simulink model "Test"  (R2018b)
settings: Solver=VariableStepAuto  StartTime=0.0  StopTime=10.0  MaxStep=0.001  MinStep=0.0001  RelTol=1e-3
model workspace (MAT data in the model file):
  Ball.radius = 0.03
  Ball.density = 1000
  Plane.length = 1
  Plane.width = 1
  Plane.depth = 0.1
  SCARA_Robot = robotics.RigidBodyTree
  SCARA_Robot.TreeInternal = robotics.manip.internal.RigidBodyTree
  SCARA_Robot.TreeInternal.NumBodies = 7
  SCARA_Robot.TreeInternal.Base = robotics.manip.internal.RigidBody
  SCARA_Robot.TreeInternal.Base.Index = 0
  SCARA_Robot.TreeInternal.Base.NameInternal = 'Base'
  SCARA_Robot.TreeInternal.Base.JointInternal = robotics.Joint
  SCARA_Robot.TreeInternal.Base.JointInternal.Type = 'fixed'
  SCARA_Robot.TreeInternal.Base.JointInternal.VelocityNumber = 0
  SCARA_Robot.TreeInternal.Base.JointInternal.PositionNumber = 0
  SCARA_Robot.TreeInternal.Base.JointInternal.MotionSubspace = [0; 0; 0; 0; 0; 0]
  SCARA_Robot.TreeInternal.Base.JointInternal.NameInternal = 'base_jnt'
  SCARA_Robot.TreeInternal.Base.ParentIndex = -1
  SCARA_Robot.TreeInternal.Base.ChildrenIndices = [1 0 0 0 0 0 1]
  SCARA_Robot.TreeInternal.Base.MassInternal = 1
  SCARA_Robot.TreeInternal.Base.CenterOfMassInternal = [0 0 0]
  SCARA_Robot.TreeInternal.Base.InertiaInternal = [1  0  0; 0  1  0; 0  0  1]
  SCARA_Robot.TreeInternal.Base.SpatialInertia = [1  0  0  0  0  0; 0  1  0  0  0  0; 0  0  1  0  0  0; 0  0  0  1  0  0; 0  0  0  0  1  0; 0  0  0  0  0  1]
  SCARA_Robot.TreeInternal.Gravity = [0 0 -9.80665]
  SCARA_Robot.TreeInternal.Bodies{1} = robotics.manip.internal.RigidBody
  SCARA_Robot.TreeInternal.Bodies{1}.Index = 1
  SCARA_Robot.TreeInternal.Bodies{1}.NameInternal = 'Body1'
  SCARA_Robot.TreeInternal.Bodies{1}.JointInternal = robotics.Joint
  SCARA_Robot.TreeInternal.Bodies{1}.JointInternal.Type = 'revolute'
  SCARA_Robot.TreeInternal.Bodies{1}.JointInternal.VelocityNumber = 1
  SCARA_Robot.TreeInternal.Bodies{1}.JointInternal.PositionNumber = 1
  SCARA_Robot.TreeInternal.Bodies{1}.JointInternal.MotionSubspace = [0; 0; 1; 0; 0; 0]
  SCARA_Robot.TreeInternal.Bodies{1}.JointInternal.InTree = 1
  SCARA_Robot.TreeInternal.Bodies{1}.JointInternal.JointToParentTransform = [1  0  0  0; 0  1  0  0; 0  0  1  0.2335; 0  0  0  1]
  SCARA_Robot.TreeInternal.Bodies{1}.JointInternal.NameInternal = 'Joint1'
  SCARA_Robot.TreeInternal.Bodies{1}.JointInternal.PositionLimitsInternal = [-3.14159265359 3.14159265359]
  SCARA_Robot.TreeInternal.Bodies{1}.JointInternal.JointAxisInternal = [0 0 1]
  SCARA_Robot.TreeInternal.Bodies{1}.ParentIndex = 0
  SCARA_Robot.TreeInternal.Bodies{1}.ChildrenIndices = [0 1]
  SCARA_Robot.TreeInternal.Bodies{1}.MassInternal = 3.12934702863
  SCARA_Robot.TreeInternal.Bodies{1}.CenterOfMassInternal = [0.108937389495 0 0.0763962080079]
  SCARA_Robot.TreeInternal.Bodies{1}.InertiaInternal = [0.0248122549552  -1.93363586828e-20  -0.0276846659585; -1.93363586828e-20  0.092692509819  4.00877355014e-19; -0.0276846659585  4.00877355014e-19  0.0776265146367]
  SCARA_Robot.TreeInternal.Bodies{1}.SpatialInertia = [0.0248122549552  -1.93363586828e-20  -0.0276846659585  0  -0.239070246528  0; -1.93363586828e-20  0.092692509819  4.00877355014e-19  0.239070246528  0  -0.340902896122; -0.0276846659585  4.00877355014e-19  0.0776265146367  0  0.340902896122  0; 0  0.239070246528  0  3.12934702863  0  0; -0.239070246528  0  0.340902896122  0  3.12934702863  0; 0  -0.340902896122  0  0  0  3.12934702863]
  SCARA_Robot.TreeInternal.Bodies{2} = robotics.manip.internal.RigidBody
  SCARA_Robot.TreeInternal.Bodies{2}.Index = 2
  SCARA_Robot.TreeInternal.Bodies{2}.NameInternal = 'Body2'
  SCARA_Robot.TreeInternal.Bodies{2}.JointInternal = robotics.Joint
  SCARA_Robot.TreeInternal.Bodies{2}.JointInternal.Type = 'revolute'
  SCARA_Robot.TreeInternal.Bodies{2}.JointInternal.VelocityNumber = 1
  SCARA_Robot.TreeInternal.Bodies{2}.JointInternal.PositionNumber = 1
  SCARA_Robot.TreeInternal.Bodies{2}.JointInternal.MotionSubspace = [0; 0; 1; 0; 0; 0]
  SCARA_Robot.TreeInternal.Bodies{2}.JointInternal.InTree = 1
  SCARA_Robot.TreeInternal.Bodies{2}.JointInternal.JointToParentTransform = [1  0  0  0.25; 0  1  0  0; 0  0  1  0.09; 0  0  0  1]
  SCARA_Robot.TreeInternal.Bodies{2}.JointInternal.NameInternal = 'Joint2'
  SCARA_Robot.TreeInternal.Bodies{2}.JointInternal.PositionLimitsInternal = [-3.14159265359 3.14159265359]
  SCARA_Robot.TreeInternal.Bodies{2}.JointInternal.JointAxisInternal = [0 0 1]
  SCARA_Robot.TreeInternal.Bodies{2}.ParentIndex = 1
  SCARA_Robot.TreeInternal.Bodies{2}.ChildrenIndices = [0 0 1]
  SCARA_Robot.TreeInternal.Bodies{2}.MassInternal = 2.8
  SCARA_Robot.TreeInternal.Bodies{2}.CenterOfMassInternal = [0.0730251626831 0 0.08]
  SCARA_Robot.TreeInternal.Bodies{2}.InertiaInternal = [0.0343024465413  9.77217250727e-20  -0.016902140627; 9.77217250727e-20  0.0618863054598  -9.17919345749e-19; -0.016902140627  -9.17919345749e-19  0.0363706015866]
  SCARA_Robot.TreeInternal.Bodies{2}.SpatialInertia = [0.0343024465413  9.77217250727e-20  -0.016902140627  0  -0.224  0; 9.77217250727e-20  0.0618863054598  -9.17919345749e-19  0.224  0  -0.204470455513; -0.016902140627  -9.17919345749e-19  0.0363706015866  0  0.204470455513  0; 0  0.224  0  2.8  0  0; -0.224  0  0.204470455513  0  2.8  0; 0  -0.204470455513  0  0  0  2.8]
  SCARA_Robot.TreeInternal.Bodies{3} = robotics.manip.internal.RigidBody
  SCARA_Robot.TreeInternal.Bodies{3}.Index = 3
  SCARA_Robot.TreeInternal.Bodies{3}.NameInternal = 'Body3'
  SCARA_Robot.TreeInternal.Bodies{3}.JointInternal = robotics.Joint
  SCARA_Robot.TreeInternal.Bodies{3}.JointInternal.Type = 'prismatic'
  SCARA_Robot.TreeInternal.Bodies{3}.JointInternal.VelocityNumber = 1
  SCARA_Robot.TreeInternal.Bodies{3}.JointInternal.PositionNumber = 1
  SCARA_Robot.TreeInternal.Bodies{3}.JointInternal.MotionSubspace = [0; 0; 0; 0; 0; 1]
  SCARA_Robot.TreeInternal.Bodies{3}.JointInternal.InTree = 1
  SCARA_Robot.TreeInternal.Bodies{3}.JointInternal.JointToParentTransform = [1  0  0  0.142; 0  1  0  -0.008; 0  0  1  0.25; 0  0  0  1]
  SCARA_Robot.TreeInternal.Bodies{3}.JointInternal.NameInternal = 'Joint3'
  SCARA_Robot.TreeInternal.Bodies{3}.JointInternal.PositionLimitsInternal = [-0.5 0.5]
  SCARA_Robot.TreeInternal.Bodies{3}.JointInternal.JointAxisInternal = [0 0 1]
  SCARA_Robot.TreeInternal.Bodies{3}.ParentIndex = 2
  SCARA_Robot.TreeInternal.Bodies{3}.ChildrenIndices = [0 0 0 1]
  SCARA_Robot.TreeInternal.Bodies{3}.MassInternal = 0.0658123859659
  SCARA_Robot.TreeInternal.Bodies{3}.CenterOfMassInternal = [0.008 0.008 -0.161652320553]
  SCARA_Robot.TreeInternal.Bodies{3}.InertiaInternal = [0.00223249562485  -4.21199270182e-06  8.51097993001e-05; -4.21199270182e-06  0.00223249562485  8.51097993001e-05; 8.51097993001e-05  8.51097993001e-05  1.08030484212e-05]
  SCARA_Robot.TreeInternal.Bodies{3}.SpatialInertia = [0.00223249562485  -4.21199270182e-06  8.51097993001e-05  0  0.0106387249125  0.000526499087728; -4.21199270182e-06  0.00223249562485  8.51097993001e-05  -0.0106387249125  0  -0.000526499087728; 8.51097993001e-05  8.51097993001e-05  1.08030484212e-05  -0.000526499087728  0.000526499087728  0; 0  -0.0106387249125  -0.000526499087728  0.0658123859659  0  0; 0.0106387249125  0  0.000526499087728  0  0.0658123859659  0; 0.000526499087728  -0.000526499087728  0  0  0  0.0658123859659]
  SCARA_Robot.TreeInternal.Bodies{4} = robotics.manip.internal.RigidBody
  SCARA_Robot.TreeInternal.Bodies{4}.Index = 4
  SCARA_Robot.TreeInternal.Bodies{4}.NameInternal = 'Body4'
  SCARA_Robot.TreeInternal.Bodies{4}.JointInternal = robotics.Joint
  SCARA_Robot.TreeInternal.Bodies{4}.JointInternal.Type = 'revolute'
  SCARA_Robot.TreeInternal.Bodies{4}.JointInternal.VelocityNumber = 1
  SCARA_Robot.TreeInternal.Bodies{4}.JointInternal.PositionNumber = 1
  SCARA_Robot.TreeInternal.Bodies{4}.JointInternal.MotionSubspace = [0; 0; 1; 0; 0; 0]
  SCARA_Robot.TreeInternal.Bodies{4}.JointInternal.InTree = 1
  SCARA_Robot.TreeInternal.Bodies{4}.JointInternal.JointToParentTransform = [1  0  0  0.008; 0  1  0  0.008; 0  0  1  -0.02; 0  0  0  1]
  SCARA_Robot.TreeInternal.Bodies{4}.JointInternal.NameInternal = 'Joint4'
  SCARA_Robot.TreeInternal.Bodies{4}.JointInternal.PositionLimitsInternal = [-3.14159265359 3.14159265359]
  SCARA_Robot.TreeInternal.Bodies{4}.JointInternal.JointAxisInternal = [0 0 1]
  SCARA_Robot.TreeInternal.Bodies{4}.ParentIndex = 3
  SCARA_Robot.TreeInternal.Bodies{4}.ChildrenIndices = [0 0 0 0 1]
  SCARA_Robot.TreeInternal.Bodies{4}.MassInternal = 0.0638828919245
  SCARA_Robot.TreeInternal.Bodies{4}.CenterOfMassInternal = [-0.000115977158264 0 -0.314685264828]
  SCARA_Robot.TreeInternal.Bodies{4}.InertiaInternal = [0.00634242429346  0  -2.33382122413e-06; 0  0.0063422366579  0; -2.33382122413e-06  0  2.29864595889e-05]
  SCARA_Robot.TreeInternal.Bodies{4}.SpatialInertia = [0.00634242429346  0  -2.33382122413e-06  0  0.0201030047632  0; 0  0.0063422366579  0  -0.0201030047632  0  7.40895626708e-06; -2.33382122413e-06  0  2.29864595889e-05  0  -7.40895626708e-06  0; 0  -0.0201030047632  0  0.0638828919245  0  0; 0.0201030047632  0  -7.40895626708e-06  0  0.0638828919245  0; 0  7.40895626708e-06  0  0  0  0.0638828919245]
  SCARA_Robot.TreeInternal.Bodies{5} = robotics.manip.internal.RigidBody
  SCARA_Robot.TreeInternal.Bodies{5}.Index = 5
  SCARA_Robot.TreeInternal.Bodies{5}.NameInternal = 'Body5'
  SCARA_Robot.TreeInternal.Bodies{5}.JointInternal = robotics.Joint
  SCARA_Robot.TreeInternal.Bodies{5}.JointInternal.Type = 'fixed'
  SCARA_Robot.TreeInternal.Bodies{5}.JointInternal.VelocityNumber = 0
  SCARA_Robot.TreeInternal.Bodies{5}.JointInternal.PositionNumber = 0
  SCARA_Robot.TreeInternal.Bodies{5}.JointInternal.MotionSubspace = [0; 0; 0; 0; 0; 0]
  SCARA_Robot.TreeInternal.Bodies{5}.JointInternal.InTree = 1
  SCARA_Robot.TreeInternal.Bodies{5}.JointInternal.JointToParentTransform = [1  0  0  -2.71050543121e-20; 0  1  0  0; 0  0  1  -0.33; 0  0  0  1]
  SCARA_Robot.TreeInternal.Bodies{5}.JointInternal.NameInternal = 'Joint5'
  SCARA_Robot.TreeInternal.Bodies{5}.ParentIndex = 4
  SCARA_Robot.TreeInternal.Bodies{5}.ChildrenIndices = [0 0 0 0 0 1]
  SCARA_Robot.TreeInternal.Bodies{5}.MassInternal = 0
  SCARA_Robot.TreeInternal.Bodies{5}.CenterOfMassInternal = [0 0 0]
  SCARA_Robot.TreeInternal.Bodies{5}.InertiaInternal = [0  0  0; 0  0  0; 0  0  0]
  SCARA_Robot.TreeInternal.Bodies{5}.SpatialInertia = [0  0  0  0  0  0; 0  0  0  0  0  0; 0  0  0  0  0  0; 0  0  0  0  0  0; 0  0  0  0  0  0; 0  0  0  0  0  0]
  SCARA_Robot.TreeInternal.Bodies{6} = robotics.manip.internal.RigidBody
  SCARA_Robot.TreeInternal.Bodies{6}.Index = 6
  SCARA_Robot.TreeInternal.Bodies{6}.NameInternal = 'Body6'
  SCARA_Robot.TreeInternal.Bodies{6}.JointInternal = robotics.Joint
  SCARA_Robot.TreeInternal.Bodies{6}.JointInternal.Type = 'fixed'
  SCARA_Robot.TreeInternal.Bodies{6}.JointInternal.VelocityNumber = 0
  SCARA_Robot.TreeInternal.Bodies{6}.JointInternal.PositionNumber = 0
  SCARA_Robot.TreeInternal.Bodies{6}.JointInternal.MotionSubspace = [0; 0; 0; 0; 0; 0]
  SCARA_Robot.TreeInternal.Bodies{6}.JointInternal.InTree = 1
  SCARA_Robot.TreeInternal.Bodies{6}.JointInternal.JointToParentTransform = [1  0  0  0; 0  1  0  0; 0  0  1  0; 0  0  0  1]
  SCARA_Robot.TreeInternal.Bodies{6}.JointInternal.NameInternal = 'Joint6'
  SCARA_Robot.TreeInternal.Bodies{6}.ParentIndex = 5
  SCARA_Robot.TreeInternal.Bodies{6}.ChildrenIndices = [0 0 0 0 0]
  SCARA_Robot.TreeInternal.Bodies{6}.MassInternal = 0.113097335529
  SCARA_Robot.TreeInternal.Bodies{6}.CenterOfMassInternal = [0 0 0]
  SCARA_Robot.TreeInternal.Bodies{6}.InertiaInternal = [4.07150407905e-05  0  0; 0  4.07150407905e-05  0; 0  0  4.07150407905e-05]
  SCARA_Robot.TreeInternal.Bodies{6}.SpatialInertia = [4.07150407905e-05  0  0  0  0  0; 0  4.07150407905e-05  0  0  0  0; 0  0  4.07150407905e-05  0  0  0; 0  0  0  0.113097335529  0  0; 0  0  0  0  0.113097335529  0; 0  0  0  0  0  0.113097335529]
  SCARA_Robot.TreeInternal.Bodies{7} = robotics.manip.internal.RigidBody
  SCARA_Robot.TreeInternal.Bodies{7}.Index = 7
  SCARA_Robot.TreeInternal.Bodies{7}.NameInternal = 'Body7'
  SCARA_Robot.TreeInternal.Bodies{7}.JointInternal = robotics.Joint
  SCARA_Robot.TreeInternal.Bodies{7}.JointInternal.Type = 'fixed'
  SCARA_Robot.TreeInternal.Bodies{7}.JointInternal.VelocityNumber = 0
  SCARA_Robot.TreeInternal.Bodies{7}.JointInternal.PositionNumber = 0
  SCARA_Robot.TreeInternal.Bodies{7}.JointInternal.MotionSubspace = [0; 0; 0; 0; 0; 0]
  SCARA_Robot.TreeInternal.Bodies{7}.JointInternal.InTree = 1
  SCARA_Robot.TreeInternal.Bodies{7}.JointInternal.JointToParentTransform = [1  0  0  0; 0  1  0  0; 0  0  1  0; 0  0  0  1]
  SCARA_Robot.TreeInternal.Bodies{7}.JointInternal.NameInternal = 'Joint7'
  SCARA_Robot.TreeInternal.Bodies{7}.ParentIndex = 0
  SCARA_Robot.TreeInternal.Bodies{7}.ChildrenIndices = [0 0 0 0 0 0]
  SCARA_Robot.TreeInternal.Bodies{7}.MassInternal = 0
  SCARA_Robot.TreeInternal.Bodies{7}.CenterOfMassInternal = [0 0 0]
  SCARA_Robot.TreeInternal.Bodies{7}.InertiaInternal = [0  0  0; 0  0  0; 0  0  0]
  SCARA_Robot.TreeInternal.Bodies{7}.SpatialInertia = [0  0  0  0  0  0; 0  0  0  0  0  0; 0  0  0  0  0  0; 0  0  0  0  0  0; 0  0  0  0  0  0; 0  0  0  0  0  0]
  SCARA_Robot.TreeInternal.NumNonFixedBodies = 4
  SCARA_Robot.TreeInternal.PositionNumber = 4
  SCARA_Robot.TreeInternal.VelocityNumber = 4
  SCARA_Robot.TreeInternal.PositionDoFMap = [1  1; 2  2; 3  3; 4  4; 0  -1; 0  -1; 0  -1]
  SCARA_Robot.TreeInternal.VelocityDoFMap = [1  1; 2  2; 3  3; 4  4; 0  -1; 0  -1; 0  -1]
  SCARA_Robot.TreeInternal.MaxNumBodies = 7
  SCARA_Robot.TreeInternal.MaxNameLength = 200
  SCARA_Robot.TreeInternal.MaxJointPositionNumber = 7
  SCARA_Robot.TreeInternal.VisualizationInfo = robotics.manip.internal.VisualizationInfo
  SCARA_Robot.TreeInternal.VisualizationInfo.ShowTag = 'DO_NOT_EDIT_DRLYM'
  SCARA_Robot.TreeInternal.DataFormatInternal = 'struct'
  Sig = Simulink.Signal
  Sig.DataType = 'auto'
  Sig.Dimensions = -1
  Sig.DimensionsMode = 'auto'
  Sig.Complexity = 'auto'
  Sig.SampleTime = -1
  Sig.SamplingMode = 'auto'
  smiData.RigidTransform(1).translation = [250 0 20]
  smiData.RigidTransform(1).angle = 3.14159265359
  smiData.RigidTransform(1).axis = [1 0 0]
  smiData.RigidTransform(1).ID = 'B[Link1-1:-:Link2-1]'
  smiData.RigidTransform(2).translation = [0 0 270]
  smiData.RigidTransform(2).angle = 3.14159265359
  smiData.RigidTransform(2).axis = [1 0 0]
  smiData.RigidTransform(2).ID = 'F[Link1-1:-:Link2-1]'
  smiData.RigidTransform(3).translation = [0 0 110]
  smiData.RigidTransform(3).angle = 0
  smiData.RigidTransform(3).axis = [0 0 0]
  smiData.RigidTransform(3).ID = 'B[Base-1:-:Link1-1]'
  smiData.RigidTransform(4).translation = [0 0 110]
  smiData.RigidTransform(4).angle = 3.14159265359
  smiData.RigidTransform(4).axis = [1 0 0]
  smiData.RigidTransform(4).ID = 'F[Base-1:-:Link1-1]'
  smiData.RigidTransform(5).translation = [142 8 20]
  smiData.RigidTransform(5).angle = 3.14159265359
  smiData.RigidTransform(5).axis = [1 0 0]
  smiData.RigidTransform(5).ID = 'B[Link2-1:-:Move-1]'
  smiData.RigidTransform(6).translation = [-8 -8 320]
  smiData.RigidTransform(6).angle = 0
  smiData.RigidTransform(6).axis = [0 0 1]
  smiData.RigidTransform(6).ID = 'F[Link2-1:-:Move-1]'
  smiData.RigidTransform(7).translation = [0 0 300]
  smiData.RigidTransform(7).angle = 3.14159265359
  smiData.RigidTransform(7).axis = [1 0 0]
  smiData.RigidTransform(7).ID = 'B[Move-1:-:Rot-1]'
  smiData.RigidTransform(8).translation = [0 0 -300]
  smiData.RigidTransform(8).angle = 0
  smiData.RigidTransform(8).axis = [0 0 0]
  smiData.RigidTransform(8).ID = 'F[Move-1:-:Rot-1]'
  smiData.RigidTransform(9).translation = [0 0 123.5]
  smiData.RigidTransform(9).angle = 0
  smiData.RigidTransform(9).axis = [0 0 0]
  smiData.RigidTransform(9).ID = 'RootGround[Base-1]'
  smiData.Solid(1).mass = 2.8
  smiData.Solid(1).CoM = [73.0251626831 0 190]
  smiData.Solid(1).MoI = [16382.4465413 29034.8171821 21439.1133089]
  smiData.Solid(1).PoI = [0 544.504186027 0]
  smiData.Solid(1).color = [0.8 0.3 0.3]
  smiData.Solid(1).opacity = 1
  smiData.Solid(1).ID = 'Link2*:*榛樿'
  smiData.Solid(2).mass = 0.0638828919245
  smiData.Solid(2).CoM = [-0.115977158264 0 15.3147351721]
  smiData.Solid(2).MoI = [16.3049156988 16.1164208702 22.9856003192]
  smiData.Solid(2).PoI = [0 -0.00233185912567 0]
  smiData.Solid(2).color = [0.3 0.8 0.3]
  smiData.Solid(2).opacity = 1
  smiData.Solid(2).ID = 'Rot*:*榛樿'
  smiData.Solid(3).mass = 7.54037730286
  smiData.Solid(3).CoM = [0 -12.2090965753 111.939248054]
  smiData.Solid(3).MoI = [67953.4260367 46975.8188154 47346.1777637]
  smiData.Solid(3).PoI = [2150.03105694 0 0]
  smiData.Solid(3).color = [1 0.5 0.8]
  smiData.Solid(3).opacity = 1
  smiData.Solid(3).ID = 'Base*:*榛樿'
  smiData.Solid(4).mass = 3.12934702863
  smiData.Solid(4).CoM = [108.937389495 0 33.6037919921]
  smiData.Solid(4).MoI = [6548.19467291 37291.3779621 40489.4430621]
  smiData.Solid(4).PoI = [0 1640.97739592 0]
  smiData.Solid(4).color = [0.3 0.3 0.5]
  smiData.Solid(4).opacity = 1
  smiData.Solid(4).ID = 'Link1*:*榛樿'
  smiData.Solid(5).mass = 0.0658123859659
  smiData.Solid(5).CoM = [0 0 158.347679447]
  smiData.Solid(5).MoI = [508.509062318 508.509062318 2.37906301758]
  smiData.Solid(5).PoI = [0 0 0]
  smiData.Solid(5).color = [1 0.3 0.3]
  smiData.Solid(5).opacity = 1
  smiData.Solid(5).ID = 'Move*:*榛樿'
  smiData.PrismaticJoint.Pz.Pos = 0
  smiData.PrismaticJoint.ID = '[Link2-1:-:Move-1]'
  smiData.RevoluteJoint(1).Rz.Pos = 0
  smiData.RevoluteJoint(1).ID = '[Link1-1:-:Link2-1]'
  smiData.RevoluteJoint(2).Rz.Pos = 0
  smiData.RevoluteJoint(2).ID = '[Base-1:-:Link1-1]'
  smiData.RevoluteJoint(3).Rz.Pos = 0
  smiData.RevoluteJoint(3).ID = '[Move-1:-:Rot-1]'
values from neighbouring files (symbols this model uses):
  smiData = struct    [SCARA_Robot_DataFile.m]
undefined symbols (not defined in the file or in its folder): X, Y, Z
libraries: sm_lib x35, nesl_utility x17, robotmaniplib x6
settings Model: Creator=wqq  LastModifiedBy=wqq

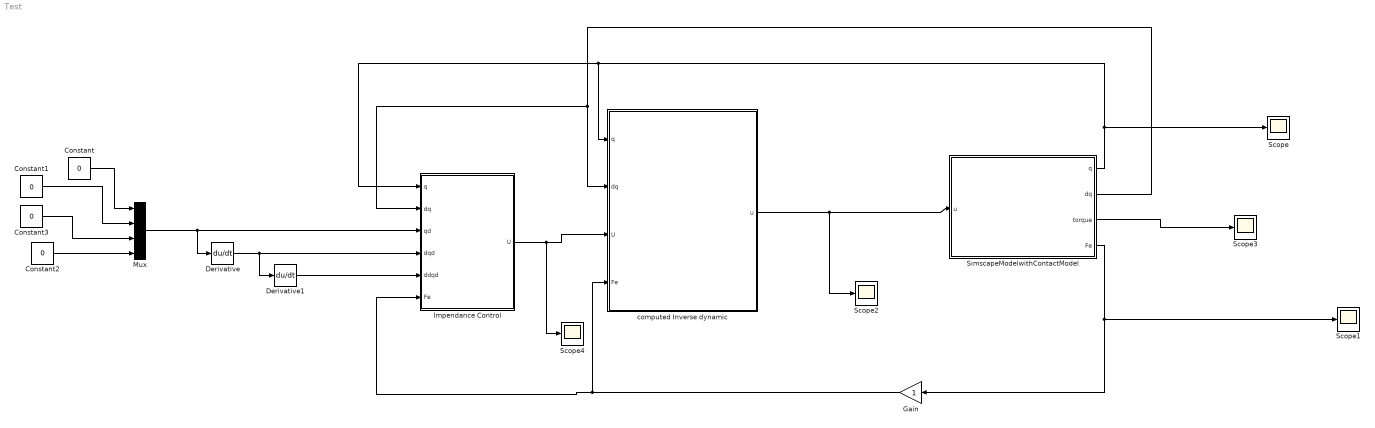
== system Test ==
  Constant{,1..3} (4 alike) : Constant  Value=0
  Derivative : Derivative
  Derivative1 : Derivative
  Gain : Gain
  Impendance Control : Subsystem
  Mux : Mux
  Scope{,1..4} (5 alike) : Scope
  SimscapeModelwithContactModel : Subsystem
  computed Inverse dynamic : Subsystem
  wires:
  SimscapeModelwithContactModel/2(dq) -> computed Inverse dynamic/2(dq), Impendance Control/2(dq)
  SimscapeModelwithContactModel/1(q) -> Scope/1, computed Inverse dynamic/1(q), Impendance Control/1(q)
  Mux/1 -> Derivative/1, Impendance Control/3(qd)
  Constant1/1 -> Mux/2
  Constant/1 -> Mux/1
  SimscapeModelwithContactModel/3(torque) -> Scope3/1
  Derivative1/1 -> Impendance Control/5(ddqd)
  SimscapeModelwithContactModel/4(Fe) -> Scope1/1, Gain/1
  Gain/1 -> computed Inverse dynamic/4(Fe), Impendance Control/6(Fe)
  Constant3/1 -> Mux/3
  computed Inverse dynamic/1(u) -> Scope2/1, SimscapeModelwithContactModel/1(u)
  Derivative/1 -> Derivative1/1, Impendance Control/4(dqd)
  Impendance Control/1(U) -> Scope4/1, computed Inverse dynamic/3(U)
  Constant2/1 -> Mux/4

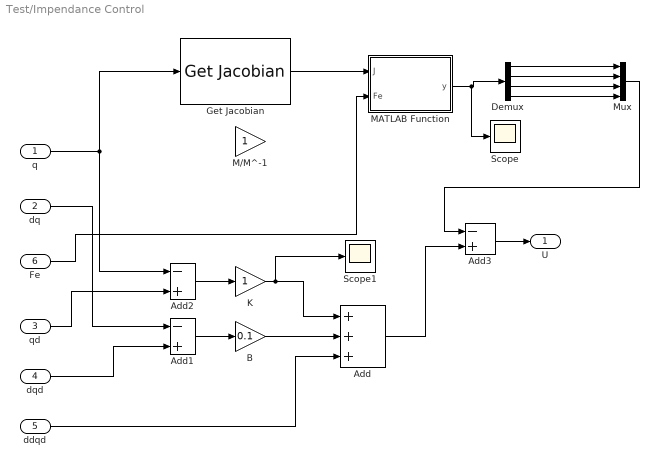
== system Test/Impendance Control ==
  q : Inport
  dq : Inport  Port=2
  qd : Inport  Port=3
  dqd : Inport  Port=4
  ddqd : Inport  Port=5
  Fe : Inport  Port=6
  Add : Sum  Inputs=+++
  Add1 : Sum  Inputs=-+
  Add2 : Sum  Inputs=-+
  Add3 : Sum  Inputs=-+
  B : Gain  Gain=0.1
  Demux : Demux
  Get Jacobian : robotmaniplib/Get Jacobian  RigidBodyTree=SCARA_Robot  EndEffector=Body7
      settings: SourceProductName=Robotics System Toolbox
  K : Gain
  M/M^-1 : Gain
  MATLAB Function : MATLAB Function  TreatAsAtomicUnit=on
  Mux : Mux
  Scope : Scope
  Scope1 : Scope
  U : Outport
  wires:
  ddqd/1 -> Add/3
  dqd/1 -> Add1/2
  dq/1 -> Add1/1
  Add1/1 -> B/1
  B/1 -> Add/2
  qd/1 -> Add2/2
  Add2/1 -> K/1
  K/1 -> Scope1/1, Add/1
  Add/1 -> Add3/2
  Add3/1 -> U/1
  q/1 -> Add2/1, Get Jacobian/1
  Get Jacobian/1 -> MATLAB Function/1(J)
  Fe/1 -> MATLAB Function/2(Fe)
  MATLAB Function/1(y) -> Scope/1, Demux/1
  Demux/1 -> Mux/1
  Demux/2 -> Mux/2
  Demux/3 -> Mux/3
  Demux/4 -> Mux/4
  Mux/1 -> Add3/1

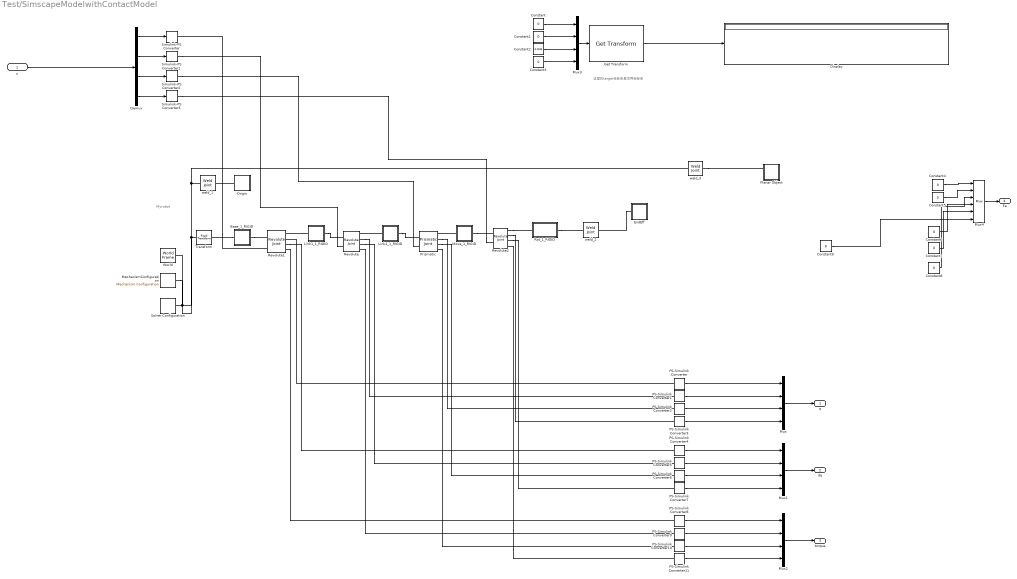
== system Test/SimscapeModelwithContactModel ==
  note: 这里的target坐标系是世界坐标系
  note: Myrobot
  u : Inport
  Base_1_RIGID : Subsystem
  Constant{,1,3..9} (9 alike) : Constant  Value=0
  Constant2 : Constant  Value=-0.2235
  Demux : Demux
  Display : Display
  EndEff : Subsystem
  Get Transform : robotmaniplib/Get Transform  RigidBodyTree=SCARA_Robot  SourceBody=Body5  TargetBody=Body7
      settings: SourceProductName=Robotics System Toolbox
  Link1_1_RIGID : Subsystem
  Link2_1_RIGID : Subsystem
  MechanismConfiguration : sm_lib/Utilities/Mechanism Configuration  UniformGravity=Constant  GravityVector=[0 0 -9.80665]  GravityUnits=m/s^2  LinearizationDelta=0.001
  Move_1_RIGID : Subsystem
  Mux{,1..3} (4 alike) : Mux
  Mux4 : Mux  Inputs=6
  Origin : Subsystem
  PS-Simulink Converter{,1..11} (12 alike) : nesl_utility/PS-Simulink Converter  PhysicalDomain=network_engine_domain  SubClassName=ps_output  LeftPortType=input  RightPortType=output  PseudoPeriodic=off  Frequencies=[]  Unit=1  AffineConversion=off
  Planar Object : Subsystem
  Prismatic : sm_lib/Joints/Prismatic Joint  SenseConstraintForce=off  SenseConstraintForceX=off  SenseConstraintForceY=off  SenseConstraintForceZ=off  SenseConstraintTorque=off  SenseConstraintTorqueX=off  SenseConstraintTorqueY=off  SenseConstraintTorqueZ=off  SenseTotalForce=off  SenseTotalForceX=off  SenseTotalForceY=off  SenseTotalForceZ=off  SenseTotalTorque=off  SenseTotalTorqueX=off  SenseTotalTorqueY=off  SenseTotalTorqueZ=off  CompositeWrenchDir=FollowerOnBase  CompositeWrenchFrame=BaseFrame  EquilibriumPosition=0  EquilibriumPositionUnits=m  SpringStiffness=0  SpringStiffnessUnits=N/m  DampingCoefficient=0  DampingCoefficientUnits=N/(m/s)  TorqueActuationMode=InputTorque  MotionActuationMode=ComputedMotion  SensePosition=on  SenseVelocity=on  SenseAcceleration=off  SenseTorqueForce=on  PositionTargetSpecify=on  PositionTargetPriority=High  PositionTargetValue=smiData.PrismaticJoint(1).Pz.Pos  PositionTargetValueUnits=m  VelocityTargetSpecify=off  VelocityTargetPriority=High  VelocityTargetValue=0  VelocityTargetValueUnits=m/s
  Revolute : sm_lib/Joints/Revolute Joint  SenseConstraintForce=off  SenseConstraintForceX=off  SenseConstraintForceY=off  SenseConstraintForceZ=off  SenseConstraintTorque=off  SenseConstraintTorqueX=off  SenseConstraintTorqueY=off  SenseConstraintTorqueZ=off  SenseTotalForce=off  SenseTotalForceX=off  SenseTotalForceY=off  SenseTotalForceZ=off  SenseTotalTorque=off  SenseTotalTorqueX=off  SenseTotalTorqueY=off  SenseTotalTorqueZ=off  CompositeWrenchDir=FollowerOnBase  CompositeWrenchFrame=BaseFrame  EquilibriumPosition=0  EquilibriumPositionUnits=rad  SpringStiffness=0  SpringStiffnessUnits=N*m/rad  DampingCoefficient=0  DampingCoefficientUnits=N*m/(rad/s)  TorqueActuationMode=InputTorque  MotionActuationMode=ComputedMotion  SensePosition=on  SenseVelocity=on  SenseAcceleration=off  SenseTorqueForce=on  PositionTargetSpecify=on  PositionTargetPriority=High  PositionTargetValue=smiData.RevoluteJoint(1).Rz.Pos  PositionTargetValueUnits=deg  VelocityTargetSpecify=off  VelocityTargetPriority=High  VelocityTargetValue=0  VelocityTargetValueUnits=deg/s
  Revolute1 : sm_lib/Joints/Revolute Joint  SenseConstraintForce=off  SenseConstraintForceX=off  SenseConstraintForceY=off  SenseConstraintForceZ=off  SenseConstraintTorque=off  SenseConstraintTorqueX=off  SenseConstraintTorqueY=off  SenseConstraintTorqueZ=off  SenseTotalForce=off  SenseTotalForceX=off  SenseTotalForceY=off  SenseTotalForceZ=off  SenseTotalTorque=off  SenseTotalTorqueX=off  SenseTotalTorqueY=off  SenseTotalTorqueZ=off  CompositeWrenchDir=FollowerOnBase  CompositeWrenchFrame=BaseFrame  EquilibriumPosition=0  EquilibriumPositionUnits=rad  SpringStiffness=0  SpringStiffnessUnits=N*m/rad  DampingCoefficient=0  DampingCoefficientUnits=N*m/(rad/s)  TorqueActuationMode=InputTorque  MotionActuationMode=ComputedMotion  SensePosition=on  SenseVelocity=on  SenseAcceleration=off  SenseTorqueForce=on  PositionTargetSpecify=on  PositionTargetPriority=High  PositionTargetValue=smiData.RevoluteJoint(2).Rz.Pos  PositionTargetValueUnits=deg  VelocityTargetSpecify=off  VelocityTargetPriority=High  VelocityTargetValue=0  VelocityTargetValueUnits=deg/s
  Revolute2 : sm_lib/Joints/Revolute Joint  SenseConstraintForce=off  SenseConstraintForceX=off  SenseConstraintForceY=off  SenseConstraintForceZ=off  SenseConstraintTorque=off  SenseConstraintTorqueX=off  SenseConstraintTorqueY=off  SenseConstraintTorqueZ=off  SenseTotalForce=off  SenseTotalForceX=off  SenseTotalForceY=off  SenseTotalForceZ=off  SenseTotalTorque=off  SenseTotalTorqueX=off  SenseTotalTorqueY=off  SenseTotalTorqueZ=off  CompositeWrenchDir=FollowerOnBase  CompositeWrenchFrame=BaseFrame  EquilibriumPosition=0  EquilibriumPositionUnits=rad  SpringStiffness=0  SpringStiffnessUnits=N*m/rad  DampingCoefficient=0  DampingCoefficientUnits=N*m/(rad/s)  TorqueActuationMode=InputTorque  MotionActuationMode=ComputedMotion  SensePosition=on  SenseVelocity=on  SenseAcceleration=off  SenseTorqueForce=on  PositionTargetSpecify=on  PositionTargetPriority=High  PositionTargetValue=smiData.RevoluteJoint(3).Rz.Pos  PositionTargetValueUnits=deg  VelocityTargetSpecify=off  VelocityTargetPriority=High  VelocityTargetValue=0  VelocityTargetValueUnits=deg/s
  Rot_1_RIGID : Subsystem
  Simulink-PS Converter{,1..3} (4 alike) : nesl_utility/Simulink-PS Converter  PhysicalDomain=network_engine_domain  SubClassName=ps_input  LeftPortType=input  RightPortType=output  PseudoPeriodic=off  Frequencies=[]  NoiseDistribution=none  NoiseParameters=[]  Unit=1  AffineConversion=off  FilteringAndDerivatives=provide  SimscapeFilterOrder=1  InputFilterTimeConstant=0.001  UdotUserProvided=0
  Solver Configuration : nesl_utility/Solver Configuration  PhysicalDomain=network_engine_domain  SubClassName=solver  LeftPortType=input  RightPortType=generic  Tones=[]  Harmonics=[]  SimulateNoise=off  Profile=off  UseLocalSampling=off  EnableSwitchedLinearOptims=on  FrequencyDomain=off  UseCCode=off  RelTol=0.001  AbsTol=1e-06  MinStep=1e-09  ToWorkspace=off  RevertToSquareIcSolve=off  NumHomotopyIterations=100  PhasorMode=off  PhasorModeNumHarmonics=1  DoDC=off  ResidualTolerance=1e-09  UseLocalSolver=off  LocalSolverChoice=NE_BACKWARD_EULER_ADVANCER  LocalSolverSampleTime=0.001  DoFixedCost=off  MaxNonlinIter=3  MaxModeIter=2  LinearAlgebra=auto  EquationFormulation=NE_TIME_EF  DelaysMemoryBudget=1024  AutomaticFiltering=on  FilteringTimeConstant=0.001  PartitionStorageMethod=AS_NEEDED  PartitionMemoryBudget=1024
  Transform : sm_lib/Frames and Transforms/Rigid Transform  TranslationMethod=Cartesian  TranslationStandardOffset=0  TranslationLengthUnit=mm  TranslationStandardAxis=+Z  TranslationCartesianOffset=smiData.RigidTransform(9).translation  TranslationROffset=0  TranslationROffsetUnits=m  TranslationZOffset=0  TranslationZOffsetUnits=m  TranslationThetaOffset=0  TranslationThetaOffsetUnits=deg  RotationMethod=ArbitraryAxis  RotationAngleUnits=rad  RotationStandardAxis=+Z  RotationAngle=smiData.RigidTransform(9).angle  RotationArbitraryAxis=smiData.RigidTransform(9).axis  FollAlignAxisA=+X  BaseAlignAxisA=+Y  FollAlignAxisB=+Y  BaseAlignAxisB=+Z  RotationSequenceAxes=FollowerAxes  RotationSequence=XYX  RotationSequenceAngles=[0 0 0]  RotationSequenceAnglesUnits=deg  RotationMatrix=[1 0 0; 0 1 0; 0 0 1]
  World : sm_lib/Frames and Transforms/World Frame
  weld_1 : sm_lib/Joints/Weld Joint  SenseConstraintForce=off  SenseConstraintForceX=off  SenseConstraintForceY=off  SenseConstraintForceZ=off  SenseConstraintTorque=off  SenseConstraintTorqueX=off  SenseConstraintTorqueY=off  SenseConstraintTorqueZ=off  SenseTotalForce=off  SenseTotalForceX=off  SenseTotalForceY=off  SenseTotalForceZ=off  SenseTotalTorque=off  SenseTotalTorqueX=off  SenseTotalTorqueY=off  SenseTotalTorqueZ=off  CompositeWrenchDir=FollowerOnBase  CompositeWrenchFrame=BaseFrame
  weld_2 : sm_lib/Joints/Weld Joint  SenseConstraintForce=off  SenseConstraintForceX=off  SenseConstraintForceY=off  SenseConstraintForceZ=off  SenseConstraintTorque=off  SenseConstraintTorqueX=off  SenseConstraintTorqueY=off  SenseConstraintTorqueZ=off  SenseTotalForce=off  SenseTotalForceX=off  SenseTotalForceY=off  SenseTotalForceZ=off  SenseTotalTorque=off  SenseTotalTorqueX=off  SenseTotalTorqueY=off  SenseTotalTorqueZ=off  CompositeWrenchDir=FollowerOnBase  CompositeWrenchFrame=BaseFrame
  weld_3 : sm_lib/Joints/Weld Joint  SenseConstraintForce=off  SenseConstraintForceX=off  SenseConstraintForceY=off  SenseConstraintForceZ=off  SenseConstraintTorque=off  SenseConstraintTorqueX=off  SenseConstraintTorqueY=off  SenseConstraintTorqueZ=off  SenseTotalForce=off  SenseTotalForceX=off  SenseTotalForceY=off  SenseTotalForceZ=off  SenseTotalTorque=off  SenseTotalTorqueX=off  SenseTotalTorqueY=off  SenseTotalTorqueZ=off  CompositeWrenchDir=FollowerOnBase  CompositeWrenchFrame=BaseFrame
  q : Outport
  dq : Outport  Port=2
  torque : Outport  Port=3
  Fe : Outport  Port=4
  wires:
  Demux/4 -> Simulink-PS Converter3/1
  Mux1/1 -> dq/1
  PS-Simulink Converter10/1 -> Mux2/3
  PS-Simulink Converter8/1 -> Mux2/1
  Demux/3 -> Simulink-PS Converter2/1
  Demux/1 -> Simulink-PS Converter/1
  PS-Simulink Converter11/1 -> Mux2/4
  PS-Simulink Converter5/1 -> Mux1/2
  PS-Simulink Converter/1 -> Mux/1
  Mux2/1 -> torque/1
  PS-Simulink Converter1/1 -> Mux/2
  Demux/2 -> Simulink-PS Converter1/1
  PS-Simulink Converter9/1 -> Mux2/2
  PS-Simulink Converter6/1 -> Mux1/3
  PS-Simulink Converter7/1 -> Mux1/4
  PS-Simulink Converter4/1 -> Mux1/1
  Mux/1 -> q/1
  PS-Simulink Converter2/1 -> Mux/3
  PS-Simulink Converter3/1 -> Mux/4
  Mux3/1 -> Get Transform/1
  Constant/1 -> Mux3/1
  Constant1/1 -> Mux3/2
  Constant2/1 -> Mux3/3
  Constant3/1 -> Mux3/4
  u/1 -> Demux/1
  Get Transform/1 -> Display/1
  Constant4/1 -> Mux4/1
  Constant5/1 -> Mux4/2
  Mux4/1 -> Fe/1
  Constant6/1 -> Mux4/4
  Constant7/1 -> Mux4/5
  Constant8/1 -> Mux4/3
  Constant9/1 -> Mux4/6
  connections:
  Revolute2/RConn3 -- PS-Simulink Converter7/LConn1
  Revolute/RConn2 -- PS-Simulink Converter1/LConn1
  Link2_1_RIGID/LConn1 -- Revolute/RConn1
  Move_1_RIGID/LConn1 -- Prismatic/RConn1
  Link1_1_RIGID/LConn1 -- Revolute1/RConn1
  Base_1_RIGID/LConn1 -- Transform/RConn1
  Revolute2/RConn2 -- PS-Simulink Converter3/LConn1
  Revolute1/LConn2 -- Simulink-PS Converter/RConn1
  Revolute1/RConn3 -- PS-Simulink Converter4/LConn1
  Simulink-PS Converter3/RConn1 -- Revolute2/LConn2
  Revolute1/RConn4 -- PS-Simulink Converter8/LConn1
  Move_1_RIGID/RConn1 -- Revolute2/LConn1
  PS-Simulink Converter/LConn1 -- Revolute1/RConn2
  Revolute/RConn4 -- PS-Simulink Converter9/LConn1
  Link2_1_RIGID/RConn1 -- Prismatic/LConn1
  Base_1_RIGID/RConn1 -- Revolute1/LConn1
  Link1_1_RIGID/RConn1 -- Revolute/LConn1
  Revolute2/RConn1 -- Rot_1_RIGID/LConn1
  Prismatic/RConn2 -- PS-Simulink Converter2/LConn1
  Revolute2/RConn4 -- PS-Simulink Converter11/LConn1
  Simulink-PS Converter2/RConn1 -- Prismatic/LConn2
  Simulink-PS Converter1/RConn1 -- Revolute/LConn2
  Revolute/RConn3 -- PS-Simulink Converter5/LConn1
  Prismatic/RConn3 -- PS-Simulink Converter6/LConn1
  Prismatic/RConn4 -- PS-Simulink Converter10/LConn1
  Rot_1_RIGID/RConn1 -- weld_2/LConn1
  EndEff/LConn1 -- weld_2/RConn1
  Origin/LConn1 -- weld_1/RConn1
  weld_1/LConn1 -- World/RConn1 -- MechanismConfiguration/RConn1 -- Solver Configuration/RConn1 -- Transform/LConn1 -- weld_3/LConn1
  weld_3/RConn1 -- Planar Object/LConn1

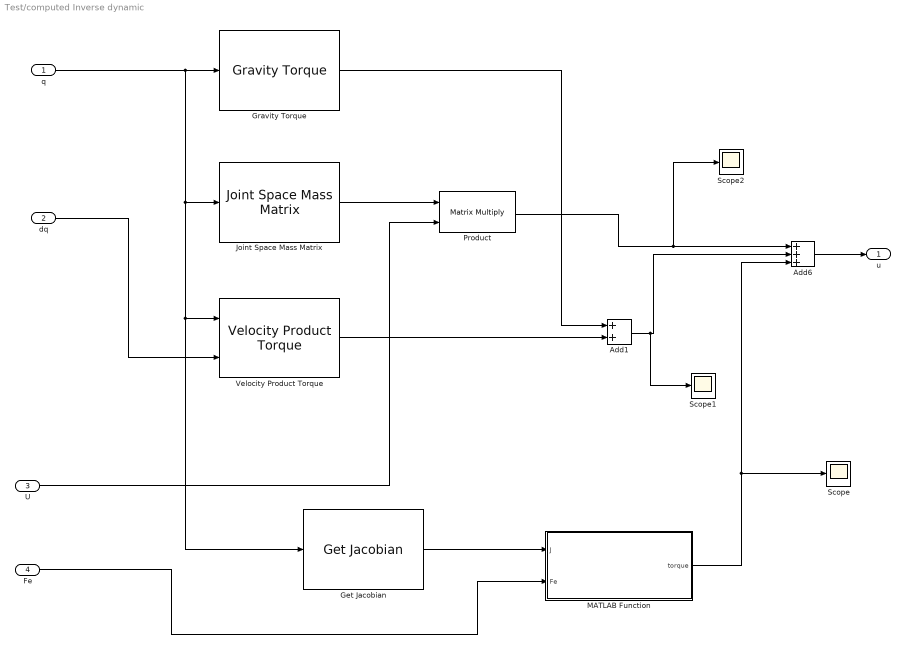
== system Test/computed Inverse dynamic ==
  q : Inport
  dq : Inport  Port=2
  U : Inport  Port=3
  Fe : Inport  Port=4
  Add1 : Sum
  Add6 : Sum  Inputs=+++
  Get Jacobian : robotmaniplib/Get Jacobian  RigidBodyTree=SCARA_Robot  EndEffector=Body7
      settings: SourceProductName=Robotics System Toolbox
  Gravity Torque : robotmaniplib/Gravity Torque  RigidBodyTree=SCARA_Robot
      settings: SourceProductName=Robotics System Toolbox
  Joint Space Mass Matrix : robotmaniplib/Joint Space Mass Matrix  RigidBodyTree=SCARA_Robot
      settings: SourceProductName=Robotics System Toolbox
  MATLAB Function : MATLAB Function  TreatAsAtomicUnit=on
  Product : Product  Multiplication=Matrix(*)
  Scope : Scope
  Scope1 : Scope
  Scope2 : Scope
  Velocity Product Torque : robotmaniplib/Velocity Product Torque  RigidBodyTree=SCARA_Robot
      settings: SourceProductName=Robotics System Toolbox
  u : Outport
  wires:
  q/1 -> Get Jacobian/1, Velocity Product Torque/1, Joint Space Mass Matrix/1, Gravity Torque/1
  dq/1 -> Velocity Product Torque/2
  Gravity Torque/1 -> Add1/1
  Joint Space Mass Matrix/1 -> Product/1
  Velocity Product Torque/1 -> Add1/2
  Add1/1 -> Scope1/1, Add6/2
  Product/1 -> Scope2/1, Add6/1
  Add6/1 -> u/1
  U/1 -> Product/2
  Get Jacobian/1 -> MATLAB Function/1(J)
  Fe/1 -> MATLAB Function/2(Fe)
  MATLAB Function/1(torque) -> Scope/1, Add6/3

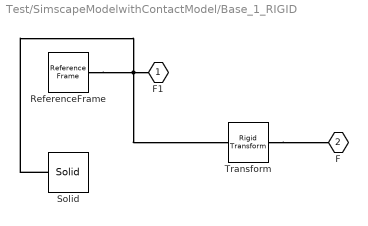
== system Test/SimscapeModelwithContactModel/Base_1_RIGID ==
  ReferenceFrame : sm_lib/Frames and Transforms/Reference Frame
  Solid : sm_lib/Body Elements/Solid  InertiaType=Custom  Mass=smiData.Solid(3).mass  MassUnits=kg  CenterOfMass=smiData.Solid(3).CoM  CenterOfMassUnits=mm  MomentsOfInertia=smiData.Solid(3).MoI  MomentsOfInertiaUnits=kg*mm^2  ProductsOfInertia=smiData.Solid(3).PoI  ProductsOfInertiaUnits=kg*mm^2  BasedOnType=Density  Density=1000  DensityUnits=kg/m^3  DoExposeReferenceFrame=off  SerializedFrames=<Frames><Frame><Id>Frame1</Id><Value><Name>F2</Name><Origin><Source>GeometricFeature</Source><FeatureName>cylindrical surface 2</FeatureName></Origin><PrimaryAxis><DefinedDirection>+Z</DefinedDirection><Source>ReferenceFrame</Source><SourceDirection>+Z</SourceDirection><FeatureName></FeatureName></PrimaryAxis><SecondaryAxis><DefinedDirection>+X</DefinedDirection><Source>ReferenceFrame</Source><SourceDirection>+X</SourceDirection><FeatureName></FeatureName></SecondaryAxis></Value></Frame></Frames>  GraphicType=FromGeometry  MarkerShape=Sphere  MarkerSize=10  GraphicVisPropType=SimpleVisualProperties  GraphicDiffuseColor=smiData.Solid(3).color  GraphicSpecularColor=[0.5 0.5 0.5 1.0]  GraphicAmbientColor=[0.15 0.15 0.15 1.0]  GraphicEmissiveColor=[0.0 0.0 0.0 1.0]  GraphicShininess=75  GraphicOpacity=smiData.Solid(3).opacity  GeometryShape=FromFile  RectangleSize=[1 1]  RectangleSizeUnits=m  BrickDimensions=[1 1 1]  BrickDimensionUnits=m  CylinderRadius=1  CylinderRadiusUnits=m  CylinderLength=1  CylinderLengthUnits=m  SphereRadius=1  SphereRadiusUnits=m  EllipsoidRadii=[1 1 1]  EllipsoidRadiiUnits=m  ExtrusionCrossSection=[1 1; -1 1; -1 -1; 1 -1]  ExtrusionCrossSectionUnits=m  ExtrusionLength=1  ExtrusionLengthUnits=m  PolygonNumSides=3  PolygonOuterRadius=1  PolygonOuterRadiusUnits=m  ExtGeomFileType=STEP  ExtGeomFileName=Base_默认_sldprt.STEP  ExtGeomFileUnits=m  RevolutionCrossSection=[1 1; 1 -1; 2 -1; 2 1]  RevolutionCrossSectionUnits=m  RevolutionExtent=Full  RevolutionAngle=180  RevolutionAngleUnits=deg
  Transform : sm_lib/Frames and Transforms/Rigid Transform  TranslationMethod=Cartesian  TranslationStandardOffset=0  TranslationLengthUnit=mm  TranslationStandardAxis=+Z  TranslationCartesianOffset=smiData.RigidTransform(3).translation  TranslationROffset=0  TranslationROffsetUnits=m  TranslationZOffset=0  TranslationZOffsetUnits=m  TranslationThetaOffset=0  TranslationThetaOffsetUnits=deg  RotationMethod=ArbitraryAxis  RotationAngleUnits=rad  RotationStandardAxis=+Z  RotationAngle=smiData.RigidTransform(3).angle  RotationArbitraryAxis=smiData.RigidTransform(3).axis  FollAlignAxisA=+X  BaseAlignAxisA=+Y  FollAlignAxisB=+Y  BaseAlignAxisB=+Z  RotationSequenceAxes=FollowerAxes  RotationSequence=XYX  RotationSequenceAngles=[0 0 0]  RotationSequenceAnglesUnits=deg  RotationMatrix=[1 0 0; 0 1 0; 0 0 1]
  F1 : PMIOPort  Side=Left
  F : PMIOPort  Port=2  Side=Right
  connections:
  ReferenceFrame/RConn1 -- Solid/LConn1 -- Transform/LConn1 -- F1/RConn1
  Transform/RConn1 -- F/RConn1

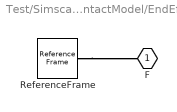
== system Test/SimscapeModelwithContactModel/EndEff ==
  ReferenceFrame : sm_lib/Frames and Transforms/Reference Frame
  F : PMIOPort  Side=Left
  connections:
  ReferenceFrame/RConn1 -- F/RConn1

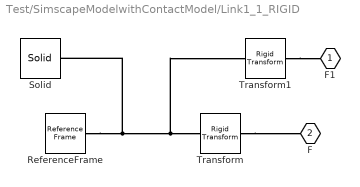
== system Test/SimscapeModelwithContactModel/Link1_1_RIGID ==
  ReferenceFrame : sm_lib/Frames and Transforms/Reference Frame
  Solid : sm_lib/Body Elements/Solid  InertiaType=Custom  Mass=smiData.Solid(4).mass  MassUnits=kg  CenterOfMass=smiData.Solid(4).CoM  CenterOfMassUnits=mm  MomentsOfInertia=smiData.Solid(4).MoI  MomentsOfInertiaUnits=kg*mm^2  ProductsOfInertia=smiData.Solid(4).PoI  ProductsOfInertiaUnits=kg*mm^2  BasedOnType=Density  Density=1000  DensityUnits=kg/m^3  DoExposeReferenceFrame=on  SerializedFrames=<Frames/>  GraphicType=FromGeometry  MarkerShape=Sphere  MarkerSize=10  GraphicVisPropType=SimpleVisualProperties  GraphicDiffuseColor=smiData.Solid(4).color  GraphicSpecularColor=[0.5 0.5 0.5 1.0]  GraphicAmbientColor=[0.15 0.15 0.15 1.0]  GraphicEmissiveColor=[0.0 0.0 0.0 1.0]  GraphicShininess=75  GraphicOpacity=smiData.Solid(4).opacity  GeometryShape=FromFile  RectangleSize=[1 1]  RectangleSizeUnits=m  BrickDimensions=[1 1 1]  BrickDimensionUnits=m  CylinderRadius=1  CylinderRadiusUnits=m  CylinderLength=1  CylinderLengthUnits=m  SphereRadius=1  SphereRadiusUnits=m  EllipsoidRadii=[1 1 1]  EllipsoidRadiiUnits=m  ExtrusionCrossSection=[1 1; -1 1; -1 -1; 1 -1]  ExtrusionCrossSectionUnits=m  ExtrusionLength=1  ExtrusionLengthUnits=m  PolygonNumSides=3  PolygonOuterRadius=1  PolygonOuterRadiusUnits=m  ExtGeomFileType=STEP  ExtGeomFileName=Link1_默认_sldprt.STEP  ExtGeomFileUnits=m  RevolutionCrossSection=[1 1; 1 -1; 2 -1; 2 1]  RevolutionCrossSectionUnits=m  RevolutionExtent=Full  RevolutionAngle=180  RevolutionAngleUnits=deg
  Transform : sm_lib/Frames and Transforms/Rigid Transform  TranslationMethod=Cartesian  TranslationStandardOffset=0  TranslationLengthUnit=mm  TranslationStandardAxis=+Z  TranslationCartesianOffset=smiData.RigidTransform(1).translation  TranslationROffset=0  TranslationROffsetUnits=m  TranslationZOffset=0  TranslationZOffsetUnits=m  TranslationThetaOffset=0  TranslationThetaOffsetUnits=deg  RotationMethod=ArbitraryAxis  RotationAngleUnits=rad  RotationStandardAxis=+Z  RotationAngle=smiData.RigidTransform(1).angle  RotationArbitraryAxis=smiData.RigidTransform(1).axis  FollAlignAxisA=+X  BaseAlignAxisA=+Y  FollAlignAxisB=+Y  BaseAlignAxisB=+Z  RotationSequenceAxes=FollowerAxes  RotationSequence=XYX  RotationSequenceAngles=[0 0 0]  RotationSequenceAnglesUnits=deg  RotationMatrix=[1 0 0; 0 1 0; 0 0 1]
  Transform1 : sm_lib/Frames and Transforms/Rigid Transform  TranslationMethod=Cartesian  TranslationStandardOffset=0  TranslationLengthUnit=mm  TranslationStandardAxis=+Z  TranslationCartesianOffset=smiData.RigidTransform(4).translation  TranslationROffset=0  TranslationROffsetUnits=m  TranslationZOffset=0  TranslationZOffsetUnits=m  TranslationThetaOffset=0  TranslationThetaOffsetUnits=deg  RotationMethod=ArbitraryAxis  RotationAngleUnits=rad  RotationStandardAxis=+Z  RotationAngle=smiData.RigidTransform(4).angle  RotationArbitraryAxis=smiData.RigidTransform(4).axis  FollAlignAxisA=+X  BaseAlignAxisA=+Y  FollAlignAxisB=+Y  BaseAlignAxisB=+Z  RotationSequenceAxes=FollowerAxes  RotationSequence=XYX  RotationSequenceAngles=[0 0 0]  RotationSequenceAnglesUnits=deg  RotationMatrix=[1 0 0; 0 1 0; 0 0 1]
  F1 : PMIOPort  Side=Left
  F : PMIOPort  Port=2  Side=Right
  connections:
  Solid/RConn1 -- Transform/LConn1 -- Transform1/LConn1 -- ReferenceFrame/RConn1
  Transform/RConn1 -- F/RConn1
  Transform1/RConn1 -- F1/RConn1

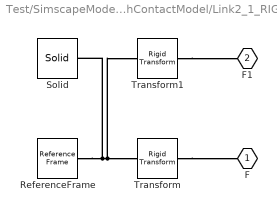
== system Test/SimscapeModelwithContactModel/Link2_1_RIGID ==
  ReferenceFrame : sm_lib/Frames and Transforms/Reference Frame
  Solid : sm_lib/Body Elements/Solid  InertiaType=Custom  Mass=smiData.Solid(1).mass  MassUnits=kg  CenterOfMass=smiData.Solid(1).CoM  CenterOfMassUnits=mm  MomentsOfInertia=smiData.Solid(1).MoI  MomentsOfInertiaUnits=kg*mm^2  ProductsOfInertia=smiData.Solid(1).PoI  ProductsOfInertiaUnits=kg*mm^2  BasedOnType=Density  Density=1000  DensityUnits=kg/m^3  DoExposeReferenceFrame=on  SerializedFrames=<Frames/>  GraphicType=FromGeometry  MarkerShape=Sphere  MarkerSize=10  GraphicVisPropType=SimpleVisualProperties  GraphicDiffuseColor=smiData.Solid(1).color  GraphicSpecularColor=[0.5 0.5 0.5 1.0]  GraphicAmbientColor=[0.15 0.15 0.15 1.0]  GraphicEmissiveColor=[0.0 0.0 0.0 1.0]  GraphicShininess=75  GraphicOpacity=smiData.Solid(1).opacity  GeometryShape=FromFile  RectangleSize=[1 1]  RectangleSizeUnits=m  BrickDimensions=[1 1 1]  BrickDimensionUnits=m  CylinderRadius=1  CylinderRadiusUnits=m  CylinderLength=1  CylinderLengthUnits=m  SphereRadius=1  SphereRadiusUnits=m  EllipsoidRadii=[1 1 1]  EllipsoidRadiiUnits=m  ExtrusionCrossSection=[1 1; -1 1; -1 -1; 1 -1]  ExtrusionCrossSectionUnits=m  ExtrusionLength=1  ExtrusionLengthUnits=m  PolygonNumSides=3  PolygonOuterRadius=1  PolygonOuterRadiusUnits=m  ExtGeomFileType=STEP  ExtGeomFileName=Link2_默认_sldprt.STEP  ExtGeomFileUnits=m  RevolutionCrossSection=[1 1; 1 -1; 2 -1; 2 1]  RevolutionCrossSectionUnits=m  RevolutionExtent=Full  RevolutionAngle=180  RevolutionAngleUnits=deg
  Transform : sm_lib/Frames and Transforms/Rigid Transform  TranslationMethod=Cartesian  TranslationStandardOffset=0  TranslationLengthUnit=mm  TranslationStandardAxis=+Z  TranslationCartesianOffset=smiData.RigidTransform(2).translation  TranslationROffset=0  TranslationROffsetUnits=m  TranslationZOffset=0  TranslationZOffsetUnits=m  TranslationThetaOffset=0  TranslationThetaOffsetUnits=deg  RotationMethod=ArbitraryAxis  RotationAngleUnits=rad  RotationStandardAxis=+Z  RotationAngle=smiData.RigidTransform(2).angle  RotationArbitraryAxis=smiData.RigidTransform(2).axis  FollAlignAxisA=+X  BaseAlignAxisA=+Y  FollAlignAxisB=+Y  BaseAlignAxisB=+Z  RotationSequenceAxes=FollowerAxes  RotationSequence=XYX  RotationSequenceAngles=[0 0 0]  RotationSequenceAnglesUnits=deg  RotationMatrix=[1 0 0; 0 1 0; 0 0 1]
  Transform1 : sm_lib/Frames and Transforms/Rigid Transform  TranslationMethod=Cartesian  TranslationStandardOffset=0  TranslationLengthUnit=mm  TranslationStandardAxis=+Z  TranslationCartesianOffset=smiData.RigidTransform(5).translation  TranslationROffset=0  TranslationROffsetUnits=m  TranslationZOffset=0  TranslationZOffsetUnits=m  TranslationThetaOffset=0  TranslationThetaOffsetUnits=deg  RotationMethod=ArbitraryAxis  RotationAngleUnits=rad  RotationStandardAxis=+Z  RotationAngle=smiData.RigidTransform(5).angle  RotationArbitraryAxis=smiData.RigidTransform(5).axis  FollAlignAxisA=+X  BaseAlignAxisA=+Y  FollAlignAxisB=+Y  BaseAlignAxisB=+Z  RotationSequenceAxes=FollowerAxes  RotationSequence=XYX  RotationSequenceAngles=[0 0 0]  RotationSequenceAnglesUnits=deg  RotationMatrix=[1 0 0; 0 1 0; 0 0 1]
  F : PMIOPort  Side=Left
  F1 : PMIOPort  Port=2  Side=Right
  connections:
  Solid/RConn1 -- ReferenceFrame/RConn1 -- Transform/LConn1 -- Transform1/LConn1
  Transform/RConn1 -- F/RConn1
  Transform1/RConn1 -- F1/RConn1

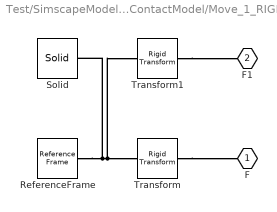
== system Test/SimscapeModelwithContactModel/Move_1_RIGID ==
  ReferenceFrame : sm_lib/Frames and Transforms/Reference Frame
  Solid : sm_lib/Body Elements/Solid  InertiaType=Custom  Mass=smiData.Solid(5).mass  MassUnits=kg  CenterOfMass=smiData.Solid(5).CoM  CenterOfMassUnits=mm  MomentsOfInertia=smiData.Solid(5).MoI  MomentsOfInertiaUnits=kg*mm^2  ProductsOfInertia=smiData.Solid(5).PoI  ProductsOfInertiaUnits=kg*mm^2  BasedOnType=Density  Density=1000  DensityUnits=kg/m^3  DoExposeReferenceFrame=on  SerializedFrames=<Frames/>  GraphicType=FromGeometry  MarkerShape=Sphere  MarkerSize=10  GraphicVisPropType=SimpleVisualProperties  GraphicDiffuseColor=smiData.Solid(5).color  GraphicSpecularColor=[0.5 0.5 0.5 1.0]  GraphicAmbientColor=[0.15 0.15 0.15 1.0]  GraphicEmissiveColor=[0.0 0.0 0.0 1.0]  GraphicShininess=75  GraphicOpacity=smiData.Solid(5).opacity  GeometryShape=FromFile  RectangleSize=[1 1]  RectangleSizeUnits=m  BrickDimensions=[1 1 1]  BrickDimensionUnits=m  CylinderRadius=1  CylinderRadiusUnits=m  CylinderLength=1  CylinderLengthUnits=m  SphereRadius=1  SphereRadiusUnits=m  EllipsoidRadii=[1 1 1]  EllipsoidRadiiUnits=m  ExtrusionCrossSection=[1 1; -1 1; -1 -1; 1 -1]  ExtrusionCrossSectionUnits=m  ExtrusionLength=1  ExtrusionLengthUnits=m  PolygonNumSides=3  PolygonOuterRadius=1  PolygonOuterRadiusUnits=m  ExtGeomFileType=STEP  ExtGeomFileName=Move_默认_sldprt.STEP  ExtGeomFileUnits=m  RevolutionCrossSection=[1 1; 1 -1; 2 -1; 2 1]  RevolutionCrossSectionUnits=m  RevolutionExtent=Full  RevolutionAngle=180  RevolutionAngleUnits=deg
  Transform : sm_lib/Frames and Transforms/Rigid Transform  TranslationMethod=Cartesian  TranslationStandardOffset=0  TranslationLengthUnit=mm  TranslationStandardAxis=+Z  TranslationCartesianOffset=smiData.RigidTransform(6).translation  TranslationROffset=0  TranslationROffsetUnits=m  TranslationZOffset=0  TranslationZOffsetUnits=m  TranslationThetaOffset=0  TranslationThetaOffsetUnits=deg  RotationMethod=ArbitraryAxis  RotationAngleUnits=rad  RotationStandardAxis=+Z  RotationAngle=smiData.RigidTransform(6).angle  RotationArbitraryAxis=smiData.RigidTransform(6).axis  FollAlignAxisA=+X  BaseAlignAxisA=+Y  FollAlignAxisB=+Y  BaseAlignAxisB=+Z  RotationSequenceAxes=FollowerAxes  RotationSequence=XYX  RotationSequenceAngles=[0 0 0]  RotationSequenceAnglesUnits=deg  RotationMatrix=[1 0 0; 0 1 0; 0 0 1]
  Transform1 : sm_lib/Frames and Transforms/Rigid Transform  TranslationMethod=Cartesian  TranslationStandardOffset=0  TranslationLengthUnit=mm  TranslationStandardAxis=+Z  TranslationCartesianOffset=smiData.RigidTransform(7).translation  TranslationROffset=0  TranslationROffsetUnits=m  TranslationZOffset=0  TranslationZOffsetUnits=m  TranslationThetaOffset=0  TranslationThetaOffsetUnits=deg  RotationMethod=ArbitraryAxis  RotationAngleUnits=rad  RotationStandardAxis=+Z  RotationAngle=0  RotationArbitraryAxis=[0 0 1]  FollAlignAxisA=+X  BaseAlignAxisA=+Y  FollAlignAxisB=+Y  BaseAlignAxisB=+Z  RotationSequenceAxes=FollowerAxes  RotationSequence=XYX  RotationSequenceAngles=[0 0 0]  RotationSequenceAnglesUnits=deg  RotationMatrix=[1 0 0; 0 1 0; 0 0 1]
  F : PMIOPort  Side=Left
  F1 : PMIOPort  Port=2  Side=Right
  connections:
  Solid/RConn1 -- ReferenceFrame/RConn1 -- Transform/LConn1 -- Transform1/LConn1
  Transform/RConn1 -- F/RConn1
  Transform1/RConn1 -- F1/RConn1

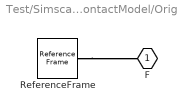
== system Test/SimscapeModelwithContactModel/Origin ==
  ReferenceFrame : sm_lib/Frames and Transforms/Reference Frame
  F : PMIOPort  Side=Left
  connections:
  ReferenceFrame/RConn1 -- F/RConn1

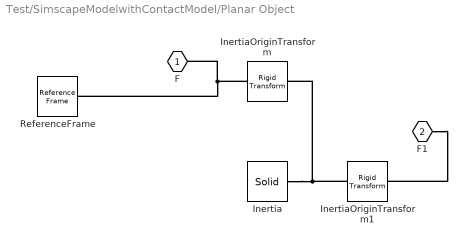
== system Test/SimscapeModelwithContactModel/Planar Object ==
  Inertia : sm_lib/Body Elements/Solid  InertiaType=Custom  Mass=1e8  MassUnits=kg  CenterOfMass=[0, 0, 0]  CenterOfMassUnits=m  MomentsOfInertia=[1e-08, 1e-08, 1e-08]  MomentsOfInertiaUnits=kg*m^2  ProductsOfInertia=[1e-08, 1e-08, 1e-08]  ProductsOfInertiaUnits=kg*m^2  BasedOnType=Density  Density=1000  DensityUnits=kg/m^3  DoExposeReferenceFrame=on  SerializedFrames=<Frames/>  GraphicType=FromGeometry  MarkerShape=Sphere  MarkerSize=10  GraphicVisPropType=SimpleVisualProperties  GraphicDiffuseColor=[0.5 0.5 0.5]  GraphicSpecularColor=[0.5 0.5 0.5 1.0]  GraphicAmbientColor=[0.15 0.15 0.15 1.0]  GraphicEmissiveColor=[0.0 0.0 0.0 1.0]  GraphicShininess=75  GraphicOpacity=1  GeometryShape=Brick  RectangleSize=[1 1]  RectangleSizeUnits=m  BrickDimensions=[0.1 1 1]  BrickDimensionUnits=m  CylinderRadius=1  CylinderRadiusUnits=m  CylinderLength=1  CylinderLengthUnits=m  SphereRadius=1  SphereRadiusUnits=m  EllipsoidRadii=[1 1 1]  EllipsoidRadiiUnits=m  ExtrusionCrossSection=[1 1; -1 1; -1 -1; 1 -1]  ExtrusionCrossSectionUnits=m  ExtrusionLength=1  ExtrusionLengthUnits=m  PolygonNumSides=3  PolygonOuterRadius=1  PolygonOuterRadiusUnits=m  ExtGeomFileType=STEP  ExtGeomFileUnits=m  RevolutionCrossSection=[1 1; 1 -1; 2 -1; 2 1]  RevolutionCrossSectionUnits=m  RevolutionExtent=Full  RevolutionAngle=180  RevolutionAngleUnits=deg
  InertiaOriginTransform : sm_lib/Frames and Transforms/Rigid Transform  TranslationMethod=Cartesian  TranslationStandardOffset=0  TranslationLengthUnit=m  TranslationStandardAxis=+Z  TranslationCartesianOffset=[0.3, 0, -0.05]  TranslationROffset=0  TranslationROffsetUnits=m  TranslationZOffset=0  TranslationZOffsetUnits=m  TranslationThetaOffset=0  TranslationThetaOffsetUnits=deg  RotationMethod=StandardAxis  RotationAngleUnits=deg  RotationStandardAxis=+Y  RotationAngle=90  RotationArbitraryAxis=[0 0 1]  FollAlignAxisA=+X  BaseAlignAxisA=+Y  FollAlignAxisB=+Y  BaseAlignAxisB=+Z  RotationSequenceAxes=BaseAxes  RotationSequence=XYZ  RotationSequenceAngles=[0, -1, 0]  RotationSequenceAnglesUnits=rad  RotationMatrix=[1 0 0; 0 -1 0; 0 0 -1]
  InertiaOriginTransform1 : sm_lib/Frames and Transforms/Rigid Transform  TranslationMethod=None  TranslationStandardOffset=0  TranslationLengthUnit=m  TranslationStandardAxis=+Z  TranslationCartesianOffset=[0.3, 0, -0.05]  TranslationROffset=0  TranslationROffsetUnits=m  TranslationZOffset=0  TranslationZOffsetUnits=m  TranslationThetaOffset=0  TranslationThetaOffsetUnits=deg  RotationMethod=RotationMatrix  RotationAngleUnits=deg  RotationStandardAxis=+Y  RotationAngle=90  RotationArbitraryAxis=[0 0 1]  FollAlignAxisA=+X  BaseAlignAxisA=+Y  FollAlignAxisB=+Y  BaseAlignAxisB=+Z  RotationSequenceAxes=BaseAxes  RotationSequence=XYZ  RotationSequenceAngles=[0, -1, 0]  RotationSequenceAnglesUnits=rad  RotationMatrix=[0 0 -1;0 -1 0;-1 0 0]
  ReferenceFrame : sm_lib/Frames and Transforms/Reference Frame
  F : PMIOPort  Side=Left
  F1 : PMIOPort  Port=2  Side=Left
  connections:
  Inertia/RConn1 -- InertiaOriginTransform1/LConn1 -- InertiaOriginTransform/RConn1
  ReferenceFrame/RConn1 -- InertiaOriginTransform/LConn1 -- F/RConn1
  F1/RConn1 -- InertiaOriginTransform1/RConn1

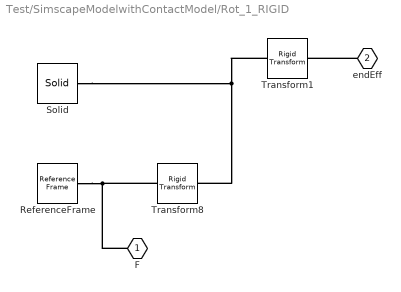
== system Test/SimscapeModelwithContactModel/Rot_1_RIGID ==
  ReferenceFrame : sm_lib/Frames and Transforms/Reference Frame
  Solid : sm_lib/Body Elements/Solid  InertiaType=Custom  Mass=smiData.Solid(2).mass  MassUnits=kg  CenterOfMass=smiData.Solid(2).CoM  CenterOfMassUnits=mm  MomentsOfInertia=smiData.Solid(2).MoI  MomentsOfInertiaUnits=kg*mm^2  ProductsOfInertia=smiData.Solid(2).PoI  ProductsOfInertiaUnits=kg*mm^2  BasedOnType=Density  Density=1000  DensityUnits=kg/m^3  DoExposeReferenceFrame=on  SerializedFrames=<Frames/>  GraphicType=FromGeometry  MarkerShape=Sphere  MarkerSize=10  GraphicVisPropType=SimpleVisualProperties  GraphicDiffuseColor=smiData.Solid(2).color  GraphicSpecularColor=[0.5 0.5 0.5 1.0]  GraphicAmbientColor=[0.15 0.15 0.15 1.0]  GraphicEmissiveColor=[0.0 0.0 0.0 1.0]  GraphicShininess=75  GraphicOpacity=smiData.Solid(2).opacity  GeometryShape=FromFile  RectangleSize=[1 1]  RectangleSizeUnits=m  BrickDimensions=[1 1 1]  BrickDimensionUnits=m  CylinderRadius=1  CylinderRadiusUnits=m  CylinderLength=1  CylinderLengthUnits=m  SphereRadius=1  SphereRadiusUnits=m  EllipsoidRadii=[1 1 1]  EllipsoidRadiiUnits=m  ExtrusionCrossSection=[1 1; -1 1; -1 -1; 1 -1]  ExtrusionCrossSectionUnits=m  ExtrusionLength=1  ExtrusionLengthUnits=m  PolygonNumSides=3  PolygonOuterRadius=1  PolygonOuterRadiusUnits=m  ExtGeomFileType=STEP  ExtGeomFileName=Rot_默认_sldprt.STEP  ExtGeomFileUnits=m  RevolutionCrossSection=[1 1; 1 -1; 2 -1; 2 1]  RevolutionCrossSectionUnits=m  RevolutionExtent=Full  RevolutionAngle=180  RevolutionAngleUnits=deg
  Transform1 : sm_lib/Frames and Transforms/Rigid Transform  TranslationMethod=StandardAxis  TranslationStandardOffset=0  TranslationLengthUnit=mm  TranslationStandardAxis=+Z  TranslationCartesianOffset=smiData.RigidTransform(8).translation  TranslationROffset=0  TranslationROffsetUnits=m  TranslationZOffset=0  TranslationZOffsetUnits=m  TranslationThetaOffset=0  TranslationThetaOffsetUnits=deg  RotationMethod=RotationSequence  RotationAngleUnits=rad  RotationStandardAxis=+Z  RotationAngle=smiData.RigidTransform(8).angle  RotationArbitraryAxis=smiData.RigidTransform(8).axis  FollAlignAxisA=+X  BaseAlignAxisA=+Y  FollAlignAxisB=+Y  BaseAlignAxisB=+Z  RotationSequenceAxes=FollowerAxes  RotationSequence=XYX  RotationSequenceAngles=[0 0 0]  RotationSequenceAnglesUnits=deg  RotationMatrix=[1 0 0; 0 -1 0; 0 0 -1]
  Transform8 : sm_lib/Frames and Transforms/Rigid Transform  TranslationMethod=Cartesian  TranslationStandardOffset=0  TranslationLengthUnit=mm  TranslationStandardAxis=+Z  TranslationCartesianOffset=[0 0 -330]  TranslationROffset=0  TranslationROffsetUnits=m  TranslationZOffset=0  TranslationZOffsetUnits=m  TranslationThetaOffset=0  TranslationThetaOffsetUnits=deg  RotationMethod=RotationSequence  RotationAngleUnits=rad  RotationStandardAxis=+Z  RotationAngle=90  RotationArbitraryAxis=[0 1 0]  FollAlignAxisA=+X  BaseAlignAxisA=+Y  FollAlignAxisB=+Y  BaseAlignAxisB=+Z  RotationSequenceAxes=FollowerAxes  RotationSequence=XYX  RotationSequenceAngles=[0 0 0]  RotationSequenceAnglesUnits=deg  RotationMatrix=[1 0 0; 0 1 0; 0 0 1]
  F : PMIOPort  Side=Left
  endEff : PMIOPort  Port=2  Side=Right
  connections:
  endEff/RConn1 -- Transform1/RConn1
  ReferenceFrame/RConn1 -- Transform8/LConn1 -- F/RConn1
  Transform1/LConn1 -- Solid/RConn1 -- Transform8/RConn1

== matlab function Test/Impendance Control/MATLAB Function ==
  data: J input; y output; Fe input
function y = Computed(J,Fe)

y = pinv(J)*Fe;

== matlab function Test/computed Inverse dynamic/MATLAB Function ==
  data: J input; torque output; Fe input
function torque = ComputedTorqueByExtroFroce(J,Fe)

torque = J'*Fe;
